simulink model "SPWM_VF_Control_3_PH_IMotr_Open"  (R2018a)
settings: Solver=ode23tb  StartTime=0.0  StopTime=0.6  MaxStep=1e-7  MinStep=1e-9  RelTol=1e-5  EnableMultiTasking=on
InitFcn:
  | t=1/4800
  | t=1/150000
  | P=4
  | F=50
  | Vdc=653
  | n=(1430*pi)/60
  | T=(4*1000)/n
libraries: powerlib x39, simulink x1
settings Model: Creator=Abid  LastModifiedBy=enes_
settings DataIOCC: LimitDataPoints=on  SaveFormat=Array
settings OptimizationCC: LifeSpan=inf
settings DebuggingCC: UnderspecifiedInitializationDetection=Classic  MergeDetectMultiDrivingBlocksExec=none  SolverPrmCheckMsg=warning  StateNameClashWarn=warning  SFUnexpectedBacktrackingDiag=warning  SFNoUnconditionalDefaultTransitionDiag=warning  SFExecutionAtInitializationDiag=none
settings HardwareCC: ProdBitPerPointer=32  ProdBitPerSizeT=32  ProdBitPerPtrDiffT=32  ProdLargestAtomicFloat=None  ProdIntDivRoundTo=Undefined  ProdEndianess=Unspecified  ProdWordSize=32  ProdHWDeviceType=32-bit Generic
settings ModelReferenceCC: PropagateSignalLabelsOutOfModel=off
settings CodeAppCC: StateflowObjectComments=on
settings GRTTargetCC: TargetLangStandard=C89/C90 (ANSI)  GeneratePreprocessorConditionals=Disable all
settings ConfigComp: CovMetricSettings=dw  CovHtmlReporting=on  CovSaveCumulativeToWorkspaceVar=on  CovSaveSingleToWorkspaceVar=on  CovExternalEMLEnable=off
settings SimscapeCC: SimscapeNormalizeSystem=off

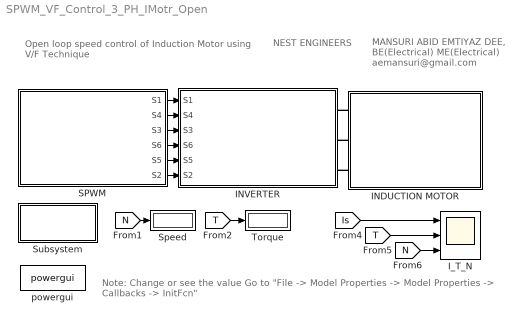
== system SPWM_VF_Control_3_PH_IMotr_Open ==
  note: Open loop speed control
      | of
      | Induction Motor using V/F Technique
  note: Note: Change or see the value
      | Go to "File -> Model Properties -> Model Properties -> Callbacks -> InitFcn"
  note: NEST
      | ENGINEERS
  note: MANSURI ABID EMTIYAZ
      | DEE, BE(Electrical)
      | ME(Electrical)
      | aemansuri@gmail.com
  INDUCTION MOTOR : Subsystem
  INVERTER : Subsystem
  I_T_N : Scope  NumInputPorts=3
  SPWM : Subsystem
  Speed : Display
  Subsystem : Subsystem
  Torque : Display
  powergui : powerlib/powergui  Priority=1  SimulationMode=Continuous  SampleTime=50e-6  frequency=60  Iterations=50  frequencyindice=0  Pbase=100e6  ErrMax=1e-4  UnitsV=kV  UnitsW=MW  buscounter=0  FunctionMessages=off  echomessages=off  EnableUseOfTLC=off  CurrentSourceSwitches=off  DisableSnubberDevices=off  DisableRonSwitches=off  DisableVfSwitches=off  DisplayEquations=off  SolverType=Tustin/Backward Euler (TBE)  Interpol=off  ExternalGateDelay=off  methode=off  Ts=100  x0status=blocks  SPID=on  SwTol=0  HookPort=off  RestoreLinks=warning  ResistiveCurrentMeasurement=off  Frange=[0:2:500]  Ylog=off  Xlog=on  ShowGrid=off  save=off  variable=ZData  structure=VF_LO_V  ZoomFFT=off  StartTime=0.5  cycles=2  DisplayStyle=1  fundamental=50  FreqAxis=on  MaxFrequency=10000  frequencyindicesteady=1  RmsSteady=1  display=off
  wires:
  SPWM/4(S6) -> INVERTER/4(S6)
  SPWM/6(S2) -> INVERTER/6(S2)
  SPWM/3(S3) -> INVERTER/3(S3)
  SPWM/1(" S1") -> INVERTER/1(S1)
  SPWM/5(S5) -> INVERTER/5(S5)
  SPWM/2(S4) -> INVERTER/2(S4)
  [N] -> Speed/1
  [T] -> Torque/1
  [Is] -> I_T_N/1
  [T] -> I_T_N/2
  [N] -> I_T_N/3
  connections:
  INDUCTION MOTOR/LConn1 -- INVERTER/RConn1
  INDUCTION MOTOR/LConn2 -- INVERTER/RConn2
  INDUCTION MOTOR/LConn3 -- INVERTER/RConn3

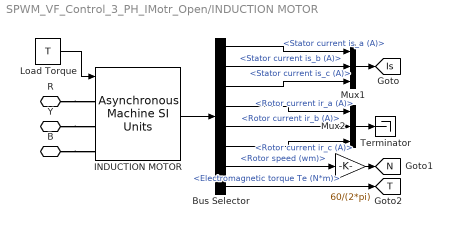
== system SPWM_VF_Control_3_PH_IMotr_Open/INDUCTION MOTOR ==
  " " : Gain  Gain=60/(2*pi)
  Bus Selector : BusSelector  OutputSignals=Stator measurements.Stator current is_a (A),Stator measurements.Stator current is_b (A),Stator measurements.Stator current is_c (A),Rotor measurements.Rotor current ir_a (A),Rotor measurements.Rotor current ir_b (A),Rotor measurements.Rotor current ir_c (A),Mechanical.Rotor speed (wm),Mechanical.Electromagnetic torque Te (N*m)
  INDUCTION MOTOR : powerlib/Machines/Asynchronous Machine SI Units  RotorType=Squirrel-cage  PresetModel="15:  5.4 HP (4KW)   400 V  50Hz 1430 RPM"  MechanicalLoad=Torque Tm  ShowDetailedParameters=on  ReferenceFrame=Rotor  Units=SI  MeasurementBus=off  NominalParameters=[4000 400 50]  Stator=[1.405 0.005839]  Rotor=[1.395 0.005839]  Cage1=[ 0.022 0.226/377]  Cage2=[ 0.022 0.226/377]  Lm=0.1722  Mechanical=[0.0131 0.002985 2]  PolePairs=2  InitialConditions=[1 0 0 0 0 0 0 0]  SimulateSaturation=off  Saturation=[14.03593122, 27.81365428, 53.79336849, 72.68890987, 97.98006896, 148.6815601, 215.7428561, 302.9841135, 420.4778367 ; 230, 322, 414, 460, 506, 552, 598, 644, 690]  LoadFlowParameters=1492000  TsPowergui=0  TsBlock=-1  IterativeModel=Trapezoidal non iterative  IterativeDiscreteModel=Trapezoidal non iterative  Pmec=0
  Load Torque : Constant  Value=T
  Mux1 : Mux  Inputs=3
  Mux2 : Mux  Inputs=3
  Terminator : Terminator
  R : PMIOPort  Side=Left
  Y : PMIOPort  Port=2  Side=Left
  B : PMIOPort  Port=3  Side=Left
  tag scope: Is=global, N=global, T=global
  wires:
  Load Torque/1 -> INDUCTION MOTOR/1
  INDUCTION MOTOR/1 -> Bus Selector/1
  Bus Selector/2 -> Mux1/2  "<Stator current is_b (A)>"
  Bus Selector/1 -> Mux1/1  "<Stator current is_a (A)>"
  Bus Selector/3 -> Mux1/3  "<Stator current is_c (A)>"
  Bus Selector/5 -> Mux2/2  "<Rotor current ir_b (A)>"
  Bus Selector/4 -> Mux2/1  "<Rotor current ir_a (A)>"
  Bus Selector/6 -> Mux2/3  "<Rotor current ir_c (A)>"
  Bus Selector/7 -> " "/1  "<Rotor speed (wm)>"
  Bus Selector/8 -> [T]  "<Electromagnetic torque Te (N*m)>"
  " "/1 -> [N]
  Mux2/1 -> Terminator/1
  Mux1/1 -> [Is]
  connections:
  R/RConn1 -- INDUCTION MOTOR/LConn1
  Y/RConn1 -- INDUCTION MOTOR/LConn2
  B/RConn1 -- INDUCTION MOTOR/LConn3

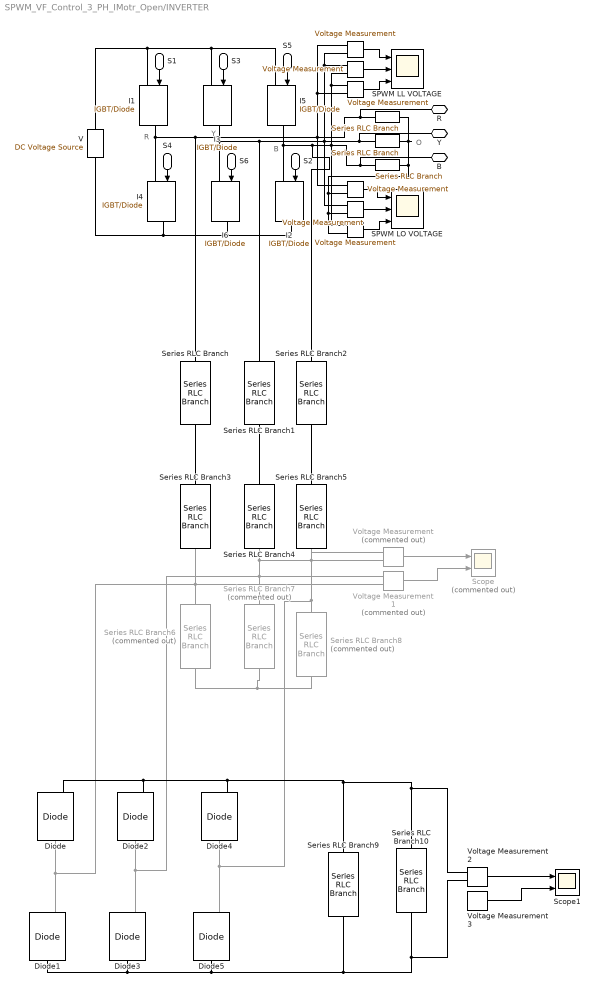
== system SPWM_VF_Control_3_PH_IMotr_Open/INVERTER ==
  note: O
  note: B
  note: Y
  note: R
  S1 : Inport
  S4 : Inport  Port=2
  S3 : Inport  Port=3
  S6 : Inport  Port=4
  S5 : Inport  Port=5
  S2 : Inport  Port=6
  " " : powerlib/Measurements/Voltage Measurement  PhasorSimulation=off  OutputType=Complex  PSBequivalent=0
  "  " : powerlib/Measurements/Voltage Measurement  PhasorSimulation=off  OutputType=Complex  PSBequivalent=0
  "   " : powerlib/Measurements/Voltage Measurement  PhasorSimulation=off  OutputType=Complex  PSBequivalent=0
  "      " : powerlib/Measurements/Voltage Measurement  PhasorSimulation=off  OutputType=Complex  PSBequivalent=0
  "         " : powerlib/Measurements/Voltage Measurement  PhasorSimulation=off  OutputType=Complex  PSBequivalent=0
  "          " : powerlib/Elements/Series RLC Branch  LConnTagsString=__new0  RConnTagsString=__new0  BranchType=R  Resistance=1  Inductance=10e-3  SetiL0=off  InitialCurrent=0  Capacitance=1e-6  Setx0=off  InitialVoltage=0  Measurements=None
  "             " : powerlib/Elements/Series RLC Branch  LConnTagsString=__new0  RConnTagsString=__new0  BranchType=R  Resistance=1  Inductance=10e-3  SetiL0=off  InitialCurrent=0  Capacitance=1e-6  Setx0=off  InitialVoltage=0  Measurements=None
  "                 " : powerlib/Elements/Series RLC Branch  LConnTagsString=__new0  RConnTagsString=__new0  BranchType=R  Resistance=1  Inductance=10e-3  SetiL0=off  InitialCurrent=0  Capacitance=1e-6  Setx0=off  InitialVoltage=0  Measurements=None
  "                  " : powerlib/Measurements/Voltage Measurement  PhasorSimulation=off  OutputType=Complex  PSBequivalent=0
  Diode{,1..5} (6 alike) : powerlib/Power Electronics/Diode  Ron=0.001  Lon=0  Vf=0.8  IC=0  UseSnubber=0  Rs=500  Cs=250e-9  Measurements=on
  I{1..6} (6 alike) : powerlib/Power Electronics/IGBT//Diode  Ron=1e-3  Rs=1e5  Cs=inf  Measurements=off
  SPWM LL VOLTAGE : Scope  NumInputPorts=3
  SPWM LO VOLTAGE : Scope  NumInputPorts=3
  Scope : Scope  Commented=on  NumInputPorts=2
  Scope1 : Scope  NumInputPorts=2
  Series RLC Branch : powerlib/Elements/Series RLC Branch  LConnTagsString=__new0  RConnTagsString=__new0  BranchType=L  Resistance=1  Inductance=82e-6  SetiL0=off  InitialCurrent=0  Capacitance=1e-6  Setx0=off  InitialVoltage=0  Measurements=None
  Series RLC Branch1 : powerlib/Elements/Series RLC Branch  LConnTagsString=__new0  RConnTagsString=__new0  BranchType=L  Resistance=1  Inductance=82e-6  SetiL0=off  InitialCurrent=0  Capacitance=1e-6  Setx0=off  InitialVoltage=0  Measurements=None
  Series RLC Branch10 : powerlib/Elements/Series RLC Branch  LConnTagsString=__new0  RConnTagsString=__new0  BranchType=R  Resistance=20  Inductance=82e-6  SetiL0=off  InitialCurrent=0  Capacitance=1/((2*pi*150e3)^2*82e-6)  Setx0=off  InitialVoltage=0  Measurements=None
  Series RLC Branch2 : powerlib/Elements/Series RLC Branch  LConnTagsString=__new0  RConnTagsString=__new0  BranchType=L  Resistance=1  Inductance=82e-6  SetiL0=off  InitialCurrent=0  Capacitance=1e-6  Setx0=off  InitialVoltage=0  Measurements=None
  Series RLC Branch3 : powerlib/Elements/Series RLC Branch  LConnTagsString=__new0  RConnTagsString=__new0  BranchType=C  Resistance=1  Inductance=82e-6  SetiL0=off  InitialCurrent=0  Capacitance=1/((2*pi*150e3)^2*82e-6)  Setx0=off  InitialVoltage=0  Measurements=None
  Series RLC Branch4 : powerlib/Elements/Series RLC Branch  LConnTagsString=__new0  RConnTagsString=__new0  BranchType=C  Resistance=1  Inductance=82e-6  SetiL0=off  InitialCurrent=0  Capacitance=1/((2*pi*150e3)^2*82e-6)  Setx0=off  InitialVoltage=0  Measurements=None
  Series RLC Branch5 : powerlib/Elements/Series RLC Branch  LConnTagsString=__new0  RConnTagsString=__new0  BranchType=C  Resistance=1  Inductance=82e-6  SetiL0=off  InitialCurrent=0  Capacitance=1/((2*pi*150e3)^2*82e-6)  Setx0=off  InitialVoltage=0  Measurements=None
  Series RLC Branch6 : powerlib/Elements/Series RLC Branch  Commented=on  LConnTagsString=__new0  RConnTagsString=__new0  BranchType=R  Resistance=20  Inductance=82e-6  SetiL0=off  InitialCurrent=0  Capacitance=1/((2*pi*150e3)^2*82e-6)  Setx0=off  InitialVoltage=0  Measurements=None
  Series RLC Branch7 : powerlib/Elements/Series RLC Branch  Commented=on  LConnTagsString=__new0  RConnTagsString=__new0  BranchType=R  Resistance=20  Inductance=82e-6  SetiL0=off  InitialCurrent=0  Capacitance=1/((2*pi*150e3)^2*82e-6)  Setx0=off  InitialVoltage=0  Measurements=None
  Series RLC Branch8 : powerlib/Elements/Series RLC Branch  Commented=on  LConnTagsString=__new0  RConnTagsString=__new0  BranchType=R  Resistance=20  Inductance=82e-6  SetiL0=off  InitialCurrent=0  Capacitance=1/((2*pi*150e3)^2*82e-6)  Setx0=off  InitialVoltage=0  Measurements=None
  Series RLC Branch9 : powerlib/Elements/Series RLC Branch  LConnTagsString=__new0  RConnTagsString=__new0  BranchType=C  Resistance=1  Inductance=82e-6  SetiL0=off  InitialCurrent=0  Capacitance=100e-6  Setx0=off  InitialVoltage=0  Measurements=None
  V : powerlib/Electrical Sources/DC Voltage Source  Amplitude=Vdc  Measurements=None
  Voltage Measurement : powerlib/Measurements/Voltage Measurement  Commented=on  PhasorSimulation=off  OutputType=Complex  PSBequivalent=0
  Voltage Measurement1 : powerlib/Measurements/Voltage Measurement  Commented=on  PhasorSimulation=off  OutputType=Complex  PSBequivalent=0
  Voltage Measurement2 : powerlib/Measurements/Voltage Measurement  PhasorSimulation=off  OutputType=Complex  PSBequivalent=0
  Voltage Measurement3 : powerlib/Measurements/Voltage Measurement  PhasorSimulation=off  OutputType=Complex  PSBequivalent=0
  "R " : PMIOPort  Side=Right
  "Y " : PMIOPort  Port=2  Side=Right
  "B " : PMIOPort  Port=3  Side=Right
  wires:
  S1/1 -> I1/1
  S3/1 -> I3/1
  S4/1 -> I4/1
  S6/1 -> I6/1
  S5/1 -> I5/1
  S2/1 -> I2/1
  "  "/1 -> SPWM LL VOLTAGE/2
  " "/1 -> SPWM LL VOLTAGE/1
  "   "/1 -> SPWM LL VOLTAGE/3
  "         "/1 -> SPWM LO VOLTAGE/2
  "      "/1 -> SPWM LO VOLTAGE/1
  "                  "/1 -> SPWM LO VOLTAGE/3
  Voltage Measurement/1 -> Scope/1
  Voltage Measurement1/1 -> Scope/2
  Voltage Measurement2/1 -> Scope1/1
  Voltage Measurement3/1 -> Scope1/2
  connections:
  V/RConn1 -- I5/LConn1 -- I3/LConn1 -- I1/LConn1
  V/LConn1 -- I2/RConn1 -- I6/RConn1 -- I4/RConn1
  I1/RConn1 -- "                 "/LConn1 -- "R "/RConn1 -- "      "/LConn1 -- "   "/LConn2 -- " "/LConn1 -- Series RLC Branch/LConn1 -- I4/LConn1
  I5/RConn1 -- Series RLC Branch2/LConn1 -- "                  "/LConn1 -- "B "/RConn1 -- "             "/LConn1 -- "   "/LConn1 -- "  "/LConn2 -- I2/LConn1
  I3/RConn1 -- Series RLC Branch1/LConn1 -- "          "/LConn1 -- "Y "/RConn1 -- "         "/LConn1 -- "  "/LConn1 -- " "/LConn2 -- I6/LConn1
  "          "/RConn1 -- "                  "/LConn2 -- "         "/LConn2 -- "      "/LConn2 -- "             "/RConn1 -- "                 "/RConn1
  Series RLC Branch3/LConn1 -- Series RLC Branch/RConn1
  Series RLC Branch4/LConn1 -- Series RLC Branch1/RConn1
  Series RLC Branch5/LConn1 -- Series RLC Branch2/RConn1
  Series RLC Branch6/RConn1 -- Series RLC Branch7/RConn1 -- Series RLC Branch8/RConn1
  Series RLC Branch6/LConn1 -- Diode1/RConn1 -- Diode/LConn1 -- Series RLC Branch3/RConn1 -- Voltage Measurement1/LConn2
  Series RLC Branch7/LConn1 -- Diode3/RConn1 -- Diode2/LConn1 -- Voltage Measurement/LConn2 -- Series RLC Branch4/RConn1 -- Voltage Measurement1/LConn1
  Series RLC Branch8/LConn1 -- Diode5/RConn1 -- Diode4/LConn1 -- Voltage Measurement/LConn1 -- Series RLC Branch5/RConn1
  Series RLC Branch9/LConn1 -- Voltage Measurement2/LConn1 -- Series RLC Branch10/LConn1 -- Diode/RConn1 -- Diode2/RConn1 -- Diode4/RConn1
  Series RLC Branch9/RConn1 -- Voltage Measurement2/LConn2 -- Series RLC Branch10/RConn1 -- Diode1/LConn1 -- Diode3/LConn1 -- Diode5/LConn1

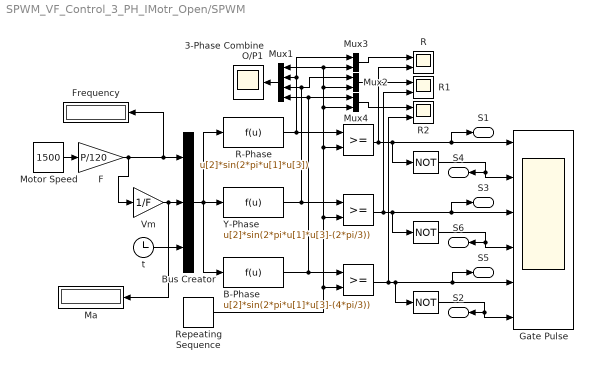
== system SPWM_VF_Control_3_PH_IMotr_Open/SPWM ==
  " " : RelationalOperator  OutDataTypeStr=boolean  RndMeth=Nearest
  "  " : RelationalOperator  OutDataTypeStr=boolean  RndMeth=Nearest
  "   " : RelationalOperator  OutDataTypeStr=boolean  RndMeth=Nearest
  "    " : Logic  Operator=NOT  AllPortsSameDT=off  OutDataTypeStr=boolean
  "     " : Logic  Operator=NOT  AllPortsSameDT=off  OutDataTypeStr=boolean
  "       " : Logic  Operator=NOT  AllPortsSameDT=off  OutDataTypeStr=boolean
  3-Phase Combine O/P1 : Scope
  B-Phase : Fcn  Expr=u[2]*sin(2*pi*u[1]*u[3]-(4*pi/3))
  Bus Creator : BusCreator  Inputs=3
  F : Gain  Gain=P/120
  Frequency : Display
  Gate Pulse : Scope  NumInputPorts=6
  Ma : Display
  Motor Speed : Constant  Value=1500
  Mux1 : Mux
  Mux2 : Mux  Inputs=2
  Mux3 : Mux  Inputs=2
  Mux4 : Mux  Inputs=2
  R : Scope  NumInputPorts=2
  R-Phase : Fcn  Expr=u[2]*sin(2*pi*u[1]*u[3])
  R1 : Scope  NumInputPorts=2
  R2 : Scope  NumInputPorts=2
  Repeating Sequence : simulink/Sources/Repeating Sequence  rep_seq_t=[0 t/2 t]  rep_seq_y=[1 -1 1]
  Vm : Gain  Gain=1/F
  Y-Phase : Fcn  Expr=u[2]*sin(2*pi*u[1]*u[3]-(2*pi/3))
  t : Clock
  " S1" : Outport
  S4 : Outport  Port=2
  S3 : Outport  Port=3
  S6 : Outport  Port=4
  S5 : Outport  Port=5
  S2 : Outport  Port=6
  wires:
  Repeating Sequence/1 -> "   "/2, "  "/2, Mux4/2, Mux3/2, Mux1/1, Mux2/2, " "/2
  " "/1 -> R/2, "    "/1, Gate Pulse/1, " S1"/1
  "    "/1 -> Gate Pulse/2, S4/1
  "     "/1 -> Gate Pulse/4, S6/1
  "   "/1 -> R2/2, "       "/1, Gate Pulse/5, S5/1
  "  "/1 -> R1/2, "     "/1, Gate Pulse/3, S3/1
  Bus Creator/1 -> R-Phase/1, Y-Phase/1, B-Phase/1
  Vm/1 -> Ma/1, Bus Creator/2
  R-Phase/1 -> Mux3/1, Mux1/2, " "/1
  Y-Phase/1 -> Mux2/1, Mux1/3, "  "/1
  B-Phase/1 -> Mux1/4, Mux4/1, "   "/1
  F/1 -> Vm/1, Frequency/1, Bus Creator/1
  t/1 -> Bus Creator/3
  Motor Speed/1 -> F/1
  "       "/1 -> Gate Pulse/6, S2/1
  Mux2/1 -> R1/1
  Mux3/1 -> R/1
  Mux4/1 -> R2/1
  Mux1/1 -> 3-Phase Combine O/P1/1

== system SPWM_VF_Control_3_PH_IMotr_Open/Subsystem ==
  note: Vph=(Vll*sqrt(2))/(sqrt(3))
      | Vph=(ma*(Vdc/2))
      | Vdc=Vph*2/ma
      | P=TW
